simulink model "dsm_l2_sim"  (R2025b)
settings: Solver=VariableStepAuto  StartTime=0.0  StopTime=510  RelTol=1e-3
values from neighbouring files (symbols this model uses):
  OLgain = 1000    [dsm_l1_plot.m]    (also in dsm_l2_plot.m)
undefined symbols (not defined in the file or in its folder): a, b, c, dspblkCoreblockFVToolHelper, g, gcbh
settings Model: Creator=dell  LastModifiedBy=dell

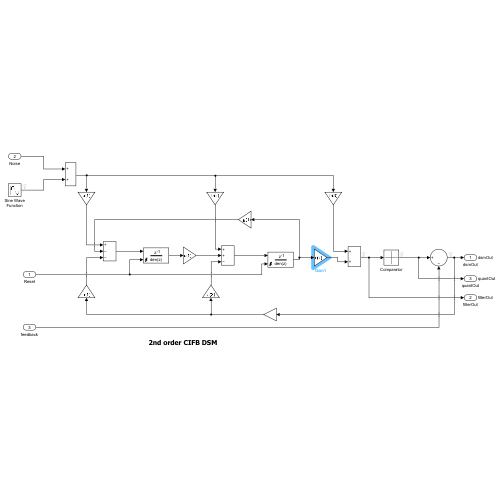
[thumbnail: Simulink's stored preview of the top-level diagram]
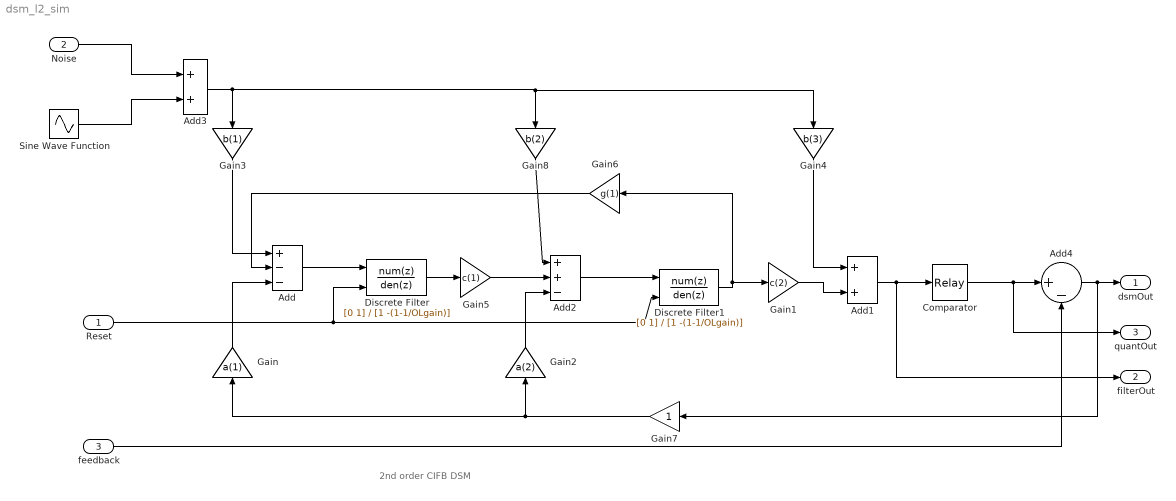
== system dsm_l2_sim ==
  note: 2nd order CIFB DSM
  Reset : Inport
  Noise : Inport  Port=2
  feedback : Inport  Port=3
  Add : Sum  Inputs=+--
  Add1 : Sum
  Add2 : Sum  Inputs=++-
  Add3 : Sum
  Add4 : Sum  Inputs=|+-
  Comparator : Relay  OnOutputValue=1.0  OffOutputValue=-1.0  ZeroCross=off
  Discrete Filter : DiscreteFilter  LoadFcn=dspblkCoreblockFVToolHelper(gcbh,'load');  Numerator=[0 1]  Denominator=[1 -(1-1/OLgain)]  ExternalReset=Rising  SampleTime=1e-06
      settings: CopyFcn=dspblkCoreblockFVToolHelper(gcbh,'copy');  DeleteFcn=dspblkCoreblockFVToolHelper(gcbh,'close');  ModelCloseFcn=dspblkCoreblockFVToolHelper(gcbh,'close');  PreSaveFcn=dspblkCoreblockFVToolHelper(gcbh,'presave');  PostSaveFcn=dspblkCoreblockFVToolHelper(gcbh,'postsave');  CloseFcn=dspblkCoreblockFVToolHelper(gcbh,'close');  InputPortMap=u0,r7
  Discrete Filter1 : DiscreteFilter  LoadFcn=dspblkCoreblockFVToolHelper(gcbh,'load');  Numerator=[0 1]  Denominator=[1 -(1-1/OLgain)]  ExternalReset=Rising  SampleTime=1e-06
      settings: CopyFcn=dspblkCoreblockFVToolHelper(gcbh,'copy');  DeleteFcn=dspblkCoreblockFVToolHelper(gcbh,'close');  ModelCloseFcn=dspblkCoreblockFVToolHelper(gcbh,'close');  PreSaveFcn=dspblkCoreblockFVToolHelper(gcbh,'presave');  PostSaveFcn=dspblkCoreblockFVToolHelper(gcbh,'postsave');  CloseFcn=dspblkCoreblockFVToolHelper(gcbh,'close');  InputPortMap=u0,r7
  Gain : Gain  Gain=a(1)
  Gain1 : Gain  Gain=c(2)
  Gain2 : Gain  Gain=a(2)
  Gain3 : Gain  Gain=b(1)
  Gain4 : Gain  Gain=b(3)  OutDataTypeStr=Inherit: Keep MSB
  Gain5 : Gain  Gain=c(1)
  Gain6 : Gain  Gain=g(1)
  Gain7 : Gain
  Gain8 : Gain  Gain=b(2)  OutDataTypeStr=Inherit: Keep MSB
  Sine Wave Function : Sin  Amplitude=0.8  Frequency=3926.9908  SampleTime=1e-06
  dsmOut : Outport  SignalName=dsmOut
  filterOut : Outport  Port=2  SignalName=filterOut
  quantOut : Outport  Port=3  SignalName=quantOut
  wires:
  Add3/1 -> Gain3/1, Gain4/1, Gain8/1
  Comparator/1 -> quantOut/1, Add4/1
  Discrete Filter/1 -> Gain5/1
  Gain8/1 -> Add2/1
  Sine Wave Function/1 -> Add3/2
  feedback/1 -> Add4/2
  Reset/1 -> Discrete Filter1/2, Discrete Filter/2
  Gain3/1 -> Add/1
  Gain7/1 -> Gain2/1, Gain/1
  Add/1 -> Discrete Filter/1
  Gain5/1 -> Add2/2
  Add4/1 -> Gain7/1, dsmOut/1
  Noise/1 -> Add3/1
  Add2/1 -> Discrete Filter1/1
  Discrete Filter1/1 -> Gain6/1, Gain1/1
  Gain2/1 -> Add2/3
  Gain/1 -> Add/3
  Gain6/1 -> Add/2
  Gain4/1 -> Add1/1
  Gain1/1 -> Add1/2
  Add1/1 -> filterOut/1, Comparator/1
